simulink model "NPO"  (R2019a)
settings: Solver=FixedStepAuto  StartTime=0.0  StopTime=300  RelTol=1e-3
InitFcn:
  | NPO_init
undefined symbols (not defined in the file or in its folder): A_w, C_w, D, K_1, K_2, K_3, K_4, M, T
settings Model: Creator=somli  LastModifiedBy=somli

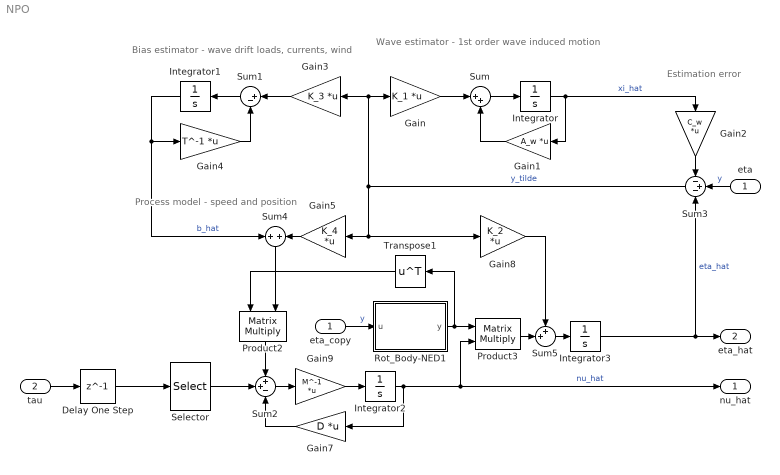
== system NPO ==
  note: Estimation error
  note: Process model - speed and position
  note: Bias estimator - wave drift loads, currents, wind
  note: Wave estimator - 1st order wave induced motion
  eta : Inport  PortDimensions=3
  tau : Inport  Port=2  PortDimensions=6
  Delay One Step : Delay  DelayLength=1
  Gain : Gain  Gain=K_1  Multiplication=Matrix(K*u)
  Gain1 : Gain  Gain=A_w  Multiplication=Matrix(K*u)
  Gain2 : Gain  Gain=C_w  Multiplication=Matrix(K*u)
  Gain3 : Gain  Gain=K_3  Multiplication=Matrix(K*u)
  Gain4 : Gain  Gain=T^-1  Multiplication=Matrix(K*u)
  Gain5 : Gain  Gain=K_4  Multiplication=Matrix(K*u)
  Gain7 : Gain  Gain=D  Multiplication=Matrix(K*u)
  Gain8 : Gain  Gain=K_2  Multiplication=Matrix(K*u)
  Gain9 : Gain  Gain=M^-1  Multiplication=Matrix(K*u)
  Integrator{,1..3} (4 alike) : Integrator
  Product2 : Product  Multiplication=Matrix(*)
  Product3 : Product  Multiplication=Matrix(*)
  Rot_Body-NED1 : MATLAB Function  TreatAsAtomicUnit=on
  Selector : Selector  InputPortWidth=6  IndexOptions=Index vector (dialog)  Indices=[1 2 6]  OutputSizes=1
  Sum : Sum  Inputs=|++
  Sum1 : Sum  Inputs=|+-
  Sum2 : Sum  Inputs=++-
  Sum3 : Sum  Inputs=-+-
  Sum4 : Sum  Inputs=+|+
  Sum5 : Sum  Inputs=++|
  Transpose1 : Math  Operator=transpose  SaturateOnIntegerOverflow=on
  eta_copy : InportShadow  PortDimensions=3
  nu_hat : Outport  PortDimensions=3
  eta_hat : Outport  Port=2  PortDimensions=3
  wires:
  Gain/1 -> Sum/1
  Sum/1 -> Integrator/1
  Gain1/1 -> Sum/2
  Integrator/1 -> Gain1/1, Gain2/1  "xi_hat"
  Gain3/1 -> Sum1/1
  Sum1/1 -> Integrator1/1
  Gain4/1 -> Sum1/2
  Integrator1/1 -> Sum4/1, Gain4/1  "b_hat"
  Product2/1 -> Sum2/1
  Sum2/1 -> Gain9/1
  Integrator2/1 -> Product3/2, nu_hat/1, Gain7/1  "nu_hat"
  Gain7/1 -> Sum2/3
  Product3/1 -> Sum5/2
  Sum5/1 -> Integrator3/1
  Sum3/1 -> Gain3/1, Gain/1, Gain8/1, Gain5/1  "y_tilde"
  Gain8/1 -> Sum5/1
  eta/1 -> Sum3/2  "y"
  Gain9/1 -> Integrator2/1
  Selector/1 -> Sum2/2
  Rot_Body-NED1/1(y) -> Product3/1, Transpose1/1
  Transpose1/1 -> Product2/1
  Integrator3/1 -> eta_hat/1, Sum3/3  "eta_hat"
  eta_copy/1 -> Rot_Body-NED1/1(u)  "y"
  Gain2/1 -> Sum3/1
  tau/1 -> Delay One Step/1
  Gain5/1 -> Sum4/2
  Sum4/1 -> Product2/2
  Delay One Step/1 -> Selector/1

== matlab function NPO/Rot_Body-NED1 ==
  data: u input; y output
function y = rot_zyx(u)
% Rzyx: Available in the MSS-toolbox
y = Rzyx(u(1), u(2), u(3));
